simulink model "induction_motor_simplified_dynamic_model_pu"  (Simulink 7.5)
settings: Solver=ode45  StartTime=0.0  StopTime=2  MaxStep=100e-6  RelTol=1e-3
InitFcn:
  | clc;
  | clear;
  | 
  | f=50;          % motor supply frequency
  | Rs=0.01;     % Stator resistance in pu
  | Rr=0.02;     % Rotor resistance in pu
  | Lls=0.10;     % Stator leakage inductance in pu
  | Llr=0.10;     % Rotor leakage inductance in pu
  | Lm=4.50;    % Magnetising reactance in pu
  | wb=2*pi*f;  % base frequency
StopFcn:
  | figure(1);
  | plot(wm,Te,'-r');
  | grid;
  | title('Torque-speed X-tics');
  | xlabel('Speed [pu]');
  | ylabel('Torque [pu]');
  | clear;
libraries: powerlib x1
Description:
  | Mathematical model of the induction machine described in the rotor flux
  | reference frame.(Per unit formulation)
  | 
  |  Electrical  system equations:
  | 
  |  Vs = Rs is + (1/wb) (dfs/dt) + wf M(pi/2) fs
  | 
  |  where the variables is, vs, and fs are 2-dimensional space vectors
  |  and M(pi/2) represents a 90 degree space rotator namely  [0 -1;1 0]
  | 
  | wf = wm + wr;
  | wr = Rr Lm/Lr (iqs / fdr)
  | 1/wb Lr/Rr (dfdr/dt) + fdr = Lm ids
  | fqr = 0
  | 
  | The flux linkage current relations:
  | fs = Ls is + Lm ir
  | fr = Lm is  + Lr ir
  | Ls= Lm + Lls;
  | Lr = Lm + Lrl
  | 
  | Mechanical system equations:
  | Te = 2H (dwm/dt) + Bm wm + Tl
  | where Te = Lm/Lr (iqs fdr)
settings Model: Creator=Abdul Rahman Kashif  LastModifiedBy=Abdul Rahman Kashif
settings DataIOCC: LimitDataPoints=off  OutputSaveName=wm,Te

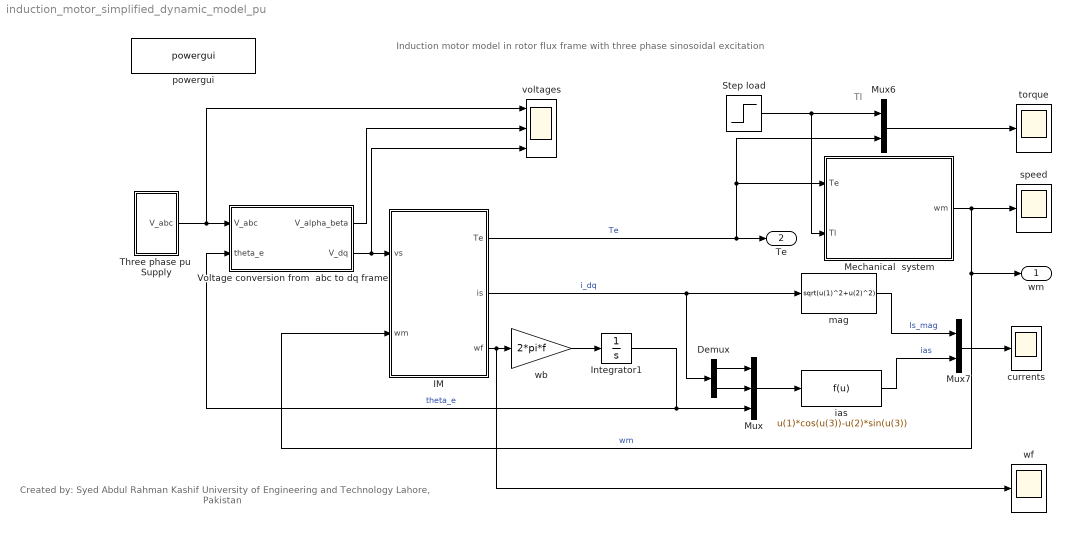
== system induction_motor_simplified_dynamic_model_pu ==
  note: Tl
  note: Induction motor model in rotor flux frame with three phase sinosoidal excitation
  note: Created by: Syed Abdul Rahman Kashif
      | University of Engineering and Technology
      | Lahore, Pakistan
  Demux : Demux  Outputs=2
  IM : Subsystem
  Integrator1 : Integrator
  Mechanical  system : Subsystem  mask{H=0.30, Bm=1e-5}
      mask prompts: H "Inertia constant [s]"; Bm "Damping coefficient [pu]"
      mask Display: disp('Mechanical\nSystem')
  Mux : Mux  Inputs=3
  Mux6 : Mux  Inputs=2
  Mux7 : Mux  Inputs=2
  Step load : Step  Time=1.5  Before=0.0  SampleTime=0
  Three phase pu  Supply : Subsystem  mask{f=f}
      mask prompts: f "Frequency"
  Voltage conversion from  abc to dq frame : Subsystem
  currents : Scope
      settings: TimeRange=2  YMin=-6  YMax=10  SaveName=ScopeData3
  ias : Fcn  Expr=u(1)*cos(u(3))-u(2)*sin(u(3))
  mag : Fcn  Expr=sqrt(u(1)^2+u(2)^2)
  powergui : powerlib/powergui  Priority=1  SystemSampleTime=-1  SimulationMode=Continuous  SampleTime=5e-6  frequency=60  SPID=off  DisableSnubberDevices=off  DisableRonSwitches=off  DisableVfSwitches=off  SwTol=0  Interpol=off  frequencyindice=50  echomessages=off  HookPort=off  DisplayEquations=off  FunctionMessages=off  EnableUseOfTLC=off  x0status=blocks  RestoreLinks=warning  ResistiveCurrentMeasurement=off  Frange=[0:2:500]  Ylog=off  Xlog=on  ShowGrid=off  save=off  variable=ZData  ZoomFFT=on  StartTime=0.0  cycles=1  DisplayStyle=1  fundamental=60  FreqAxis=off  MaxFrequency=1000  frequencyindicesteady=1  RmsSteady=1  display=off  Ts=0  methode=off
  speed : Scope
      settings: TimeRange=2  YMin=0  YMax=1.4  SaveName=wm  MaxDataPoints=20000  Decimation=20
  torque : Scope
      settings: TimeRange=2  YMin=-3  YMax=3  MaxDataPoints=20000  Decimation=20
  voltages : Scope  NumInputPorts=3
      settings: TimeRange=0.02  YMin=-1.5~-1.5~-0.5  YMax=1.5~1.5~1.5  SaveName=ScopeData2
  wb : Gain  Gain=2*pi*f  ParameterDataType=sfix(16)  ParameterScaling=2^0  OutDataType=sfix(16)  OutScaling=2^0  SaturateOnIntegerOverflow=on  OutDataTypeStr=Inherit: Same as input  ParamDataTypeStr=Inherit: Same as input
  wf : Scope
      settings: TimeRange=2  YMin=-2.5  YMax=2  MaxDataPoints=20000  Decimation=20
  wm : Outport
  Te : Outport  Port=2
  wires:
  Mux6/1 -> torque/1
  Mechanical  system/1(wm) -> speed/1, wm/1, IM/2(wm)  "wm"
  Voltage conversion from  abc to dq frame/2(V_dq) -> IM/1(vs), voltages/3
  Step load/1 -> Mux6/1, Mechanical  system/2(Tl)
  Demux/1 -> Mux/1
  Demux/2 -> Mux/2
  Mux/1 -> ias/1
  ias/1 -> Mux7/2  "ias"
  mag/1 -> Mux7/1  "Is_mag"
  Mux7/1 -> currents/1
  IM/2(is) -> mag/1, Demux/1  "i_dq"
  IM/1(Te) -> Te/1, Mux6/2, Mechanical  system/1(Te)  "Te"
  wb/1 -> Integrator1/1
  IM/3(wf) -> wb/1, wf/1
  Integrator1/1 -> Mux/3, Voltage conversion from  abc to dq frame/2(theta_e)  "theta_e"
  Voltage conversion from  abc to dq frame/1(V_alpha_beta) -> voltages/2
  Three phase pu  Supply/1(V_abc) -> voltages/1, Voltage conversion from  abc to dq frame/1(V_abc)

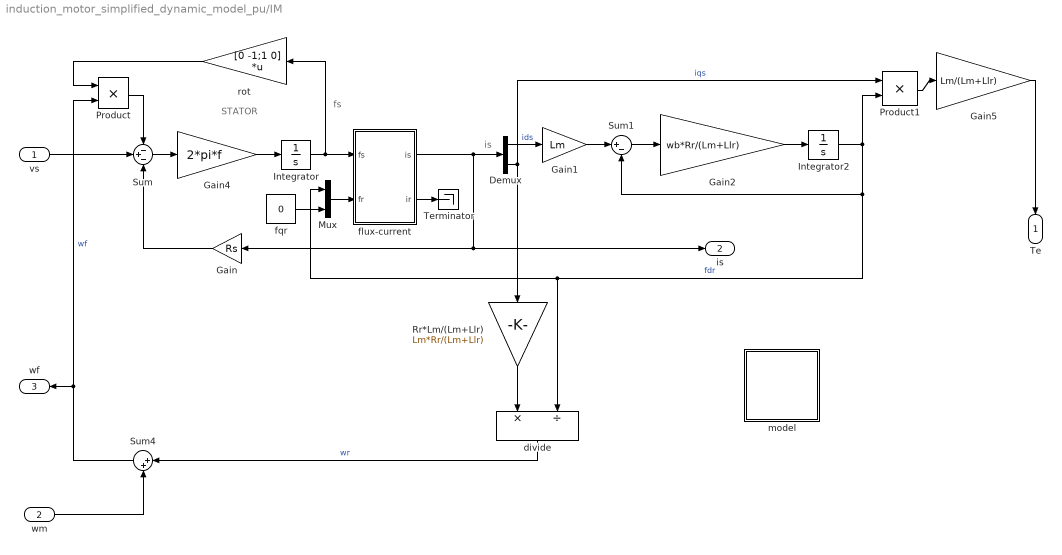
== system induction_motor_simplified_dynamic_model_pu/IM ==
  note: STATOR
  note: fs
  note: is
  vs : Inport  OutDataType=sfix(16)  OutScaling=2^0
  wm : Inport  Port=2  OutDataType=sfix(16)  OutScaling=2^0
  Demux : Demux  Outputs=2
  Gain : Gain  Gain=Rs  ParameterDataType=sfix(16)  ParameterScaling=2^0  OutDataType=sfix(16)  OutScaling=2^0  SaturateOnIntegerOverflow=on  OutDataTypeStr=Inherit: Same as input  ParamDataTypeStr=Inherit: Same as input
  Gain1 : Gain  Gain=Lm  ParameterDataType=sfix(16)  ParameterScaling=2^0  OutDataType=sfix(16)  OutScaling=2^0  SaturateOnIntegerOverflow=on  OutDataTypeStr=Inherit: Same as input  ParamDataTypeStr=Inherit: Same as input
  Gain2 : Gain  Gain=wb*Rr/(Lm+Llr)  ParameterDataType=sfix(16)  ParameterScaling=2^0  OutDataType=sfix(16)  OutScaling=2^0  SaturateOnIntegerOverflow=on  OutDataTypeStr=Inherit: Same as input  ParamDataTypeStr=Inherit: Same as input
  Gain4 : Gain  Gain=2*pi*f  ParameterDataType=sfix(16)  ParameterScaling=2^0  OutDataType=sfix(16)  OutScaling=2^0  SaturateOnIntegerOverflow=on  OutDataTypeStr=Inherit: Same as input  ParamDataTypeStr=Inherit: Same as input
  Gain5 : Gain  Gain=Lm/(Lm+Llr)  ParameterDataType=sfix(16)  ParameterScaling=2^0  OutDataType=sfix(16)  OutScaling=2^0  SaturateOnIntegerOverflow=on  OutDataTypeStr=Inherit: Same as input  ParamDataTypeStr=Inherit: Same as input
  Integrator : Integrator  InitialCondition=[0 0]
  Integrator2 : Integrator  InitialCondition=1e-5
  Mux : Mux  Inputs=2
  Product : Product  OutDataType=sfix(16)  OutScaling=2^0  SaturateOnIntegerOverflow=on  InputSameDT=on  OutDataTypeStr=Inherit: Same as first input
  Product1 : Product  OutDataType=sfix(16)  OutScaling=2^0  SaturateOnIntegerOverflow=on  InputSameDT=on  OutDataTypeStr=Inherit: Same as first input
  Rr*Lm/(Lm+Llr) : Gain  Gain=Lm*Rr/(Lm+Llr)  ParameterDataType=sfix(16)  ParameterScaling=2^0  OutDataType=sfix(16)  OutScaling=2^0  SaturateOnIntegerOverflow=on  OutDataTypeStr=Inherit: Same as input  ParamDataTypeStr=Inherit: Same as input
  Sum : Sum  Inputs=-+-  OutDataType=sfix(16)  OutScaling=2^0  SaturateOnIntegerOverflow=on  InputSameDT=on  OutDataTypeStr=Inherit: Same as first input
  Sum1 : Sum  Inputs=|+-  OutDataType=sfix(16)  OutScaling=2^0  SaturateOnIntegerOverflow=on  InputSameDT=on  OutDataTypeStr=Inherit: Same as first input
  Sum4 : Sum  Inputs=|++  OutDataType=sfix(16)  OutScaling=2^0  SaturateOnIntegerOverflow=on  InputSameDT=on  OutDataTypeStr=Inherit: Same as first input
  Terminator : Terminator
  divide : Product  Inputs=*/  OutDataType=sfix(16)  OutScaling=2^0  SaturateOnIntegerOverflow=on  InputSameDT=on  OutDataTypeStr=Inherit: Same as first input
  flux-current : Subsystem
  fqr : Constant  Value=0  OutDataType=sfix(16)  OutScaling=2^0
  model : Subsystem
      mask Display:
      | plot(-1.5,-1.5,1.5,1.5,cos(0:.01:7),sin(0:.01:7) )
      | disp('MODEL')
  rot : Gain  Gain=[0 -1;1 0]  Multiplication=Matrix(K*u)  ParameterDataType=sfix(16)  ParameterScaling=2^0  OutDataType=sfix(16)  OutScaling=2^0  SaturateOnIntegerOverflow=on  OutDataTypeStr=Inherit: Same as input  ParamDataTypeStr=Inherit: Same as input
  Te : Outport
  is : Outport  Port=2
  wf : Outport  Port=3
  wires:
  Gain/1 -> Sum/3
  Integrator/1 -> flux-current/1(fs), rot/1
  Product/1 -> Sum/1
  rot/1 -> Product/1
  Sum/1 -> Gain4/1
  Gain4/1 -> Integrator/1
  flux-current/1(is) -> Gain/1, is/1, Demux/1
  vs/1 -> Sum/2
  wm/1 -> Sum4/2
  Rr*Lm/(Lm+Llr)/1 -> divide/1
  Demux/1 -> Gain1/1  "ids"
  Sum4/1 -> Product/2, wf/1  "wf"
  divide/1 -> Sum4/1  "wr"
  fqr/1 -> Mux/2
  Demux/2 -> Rr*Lm/(Lm+Llr)/1, Product1/1  "iqs"
  Gain1/1 -> Sum1/1
  Sum1/1 -> Gain2/1
  Gain2/1 -> Integrator2/1
  Integrator2/1 -> divide/2, Mux/1, Sum1/2, Product1/2  "fdr"
  Product1/1 -> Gain5/1
  Gain5/1 -> Te/1
  Mux/1 -> flux-current/2(fr)
  flux-current/2(ir) -> Terminator/1

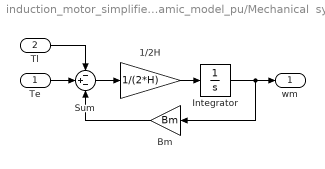
== system induction_motor_simplified_dynamic_model_pu/Mechanical  system ==
  Te : Inport  OutDataType=sfix(16)  OutScaling=2^0
  Tl : Inport  Port=2  OutDataType=sfix(16)  OutScaling=2^0
  1/2H : Gain  Gain=1/(2*H)  ParameterDataType=sfix(16)  ParameterScaling=2^0  OutDataType=sfix(16)  OutScaling=2^0  SaturateOnIntegerOverflow=on  OutDataTypeStr=Inherit: Same as input  ParamDataTypeStr=Inherit: Same as input
  Bm : Gain  Gain=Bm  ParameterDataType=sfix(16)  ParameterScaling=2^0  OutDataType=sfix(16)  OutScaling=2^0  SaturateOnIntegerOverflow=on  OutDataTypeStr=Inherit: Same as input  ParamDataTypeStr=Inherit: Same as input
  Integrator : Integrator
  Sum : Sum  Inputs=-+-  OutDataType=sfix(16)  OutScaling=2^0  SaturateOnIntegerOverflow=on  InputSameDT=on  OutDataTypeStr=Inherit: Same as first input
  wm : Outport
  wires:
  1/2H/1 -> Integrator/1
  Sum/1 -> 1/2H/1
  Bm/1 -> Sum/3
  Integrator/1 -> Bm/1, wm/1
  Te/1 -> Sum/2
  Tl/1 -> Sum/1

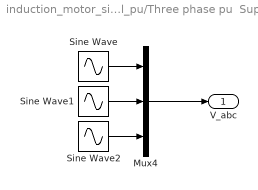
== system induction_motor_simplified_dynamic_model_pu/Three phase pu  Supply ==
  Mux4 : Mux  Inputs=3
  Sine Wave : Sin  Amplitude=1  Bias=0  Frequency=2*pi*f  Phase=pi  Samples=10  SampleTime=0  Offset=0
  Sine Wave1 : Sin  Amplitude=1  Bias=0  Frequency=2*pi*f  Phase=pi-2*pi/3  Samples=10  SampleTime=0  Offset=0
  Sine Wave2 : Sin  Amplitude=1  Bias=0  Frequency=2*pi*f  Phase=pi+2*pi/3  Samples=10  SampleTime=0  Offset=0
  V_abc : Outport
  wires:
  Sine Wave/1 -> Mux4/1
  Sine Wave1/1 -> Mux4/2
  Sine Wave2/1 -> Mux4/3
  Mux4/1 -> V_abc/1

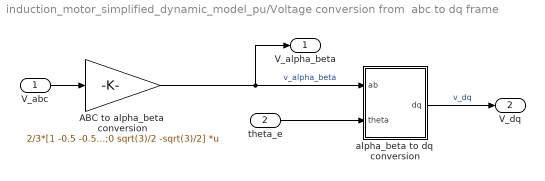
== system induction_motor_simplified_dynamic_model_pu/Voltage conversion from  abc to dq frame ==
  V_abc : Inport
  theta_e : Inport  Port=2
  ABC to alpha_beta  conversion : Gain  Gain=2/3*[1 -0.5 -0.5;0 sqrt(3)/2 -sqrt(3)/2]  Multiplication=Matrix(K*u)  ParameterDataType=sfix(16)  ParameterScaling=2^0  OutDataType=sfix(16)  OutScaling=2^0  SaturateOnIntegerOverflow=on  OutDataTypeStr=Inherit: Same as input  ParamDataTypeStr=Inherit: Same as input
  alpha_beta to dq  conversion : Subsystem
  V_alpha_beta : Outport
  V_dq : Outport  Port=2
  wires:
  ABC to alpha_beta  conversion/1 -> alpha_beta to dq  conversion/1(ab), V_alpha_beta/1  "v_alpha_beta"
  V_abc/1 -> ABC to alpha_beta  conversion/1
  theta_e/1 -> alpha_beta to dq  conversion/2(theta)
  alpha_beta to dq  conversion/1(dq) -> V_dq/1  "v_dq"

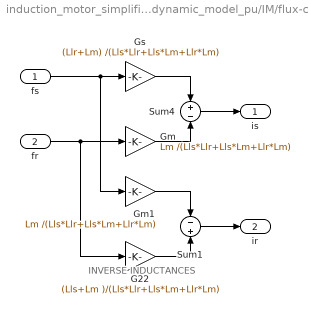
== system induction_motor_simplified_dynamic_model_pu/IM/flux-current ==
  note: INVERSE INDUCTANCES
  fs : Inport  OutDataType=sfix(16)  OutScaling=2^0
  fr : Inport  Port=2  OutDataType=sfix(16)  OutScaling=2^0
  G22 : Gain  Gain=(Lls+Lm )/(Lls*Llr+Lls*Lm+Llr*Lm)  ParameterDataType=sfix(16)  ParameterScaling=2^0  OutDataType=sfix(16)  OutScaling=2^0  SaturateOnIntegerOverflow=on  OutDataTypeStr=Inherit: Same as input  ParamDataTypeStr=Inherit: Same as input
  Gm : Gain  Gain=Lm /(Lls*Llr+Lls*Lm+Llr*Lm)  ParameterDataType=sfix(16)  ParameterScaling=2^0  OutDataType=sfix(16)  OutScaling=2^0  SaturateOnIntegerOverflow=on  OutDataTypeStr=Inherit: Same as input  ParamDataTypeStr=Inherit: Same as input
  Gm1 : Gain  Gain=Lm /(Lls*Llr+Lls*Lm+Llr*Lm)  ParameterDataType=sfix(16)  ParameterScaling=2^0  OutDataType=sfix(16)  OutScaling=2^0  SaturateOnIntegerOverflow=on  OutDataTypeStr=Inherit: Same as input  ParamDataTypeStr=Inherit: Same as input
  Gs : Gain  Gain=(Llr+Lm) /(Lls*Llr+Lls*Lm+Llr*Lm)  ParameterDataType=sfix(16)  ParameterScaling=2^0  OutDataType=sfix(16)  OutScaling=2^0  SaturateOnIntegerOverflow=on  OutDataTypeStr=Inherit: Same as input  ParamDataTypeStr=Inherit: Same as input
  Sum1 : Sum  Inputs=-+  OutDataType=sfix(16)  OutScaling=2^0  SaturateOnIntegerOverflow=on  InputSameDT=on  OutDataTypeStr=Inherit: Same as first input
  Sum4 : Sum  Inputs=+-  OutDataType=sfix(16)  OutScaling=2^0  SaturateOnIntegerOverflow=on  InputSameDT=on  OutDataTypeStr=Inherit: Same as first input
  is : Outport
  ir : Outport  Port=2
  wires:
  fs/1 -> Gs/1, Gm1/1
  Gs/1 -> Sum4/1
  fr/1 -> Gm/1, G22/1
  Gm/1 -> Sum4/2
  Sum4/1 -> is/1
  Gm1/1 -> Sum1/1
  G22/1 -> Sum1/2
  Sum1/1 -> ir/1

== system induction_motor_simplified_dynamic_model_pu/IM/model ==
  note: Mathematical model of the induction machine
      | described in the rotor flux reference frame.
      | (Per unit formulation)
  note: Electrical  system equations:
      |             vs = Rs is + 1/wo (dfs/dt) + wf M(pi/2) fs
      |                   where the variables is, vs, and fs are 2-dimensional space vectors
      |                   and M(pi/2) represents a 90o space rotator namely  [0 -1;1 0]
      |             wf = wm + wr;  wr = Rr Lm/Lr (iqs / fdr)
      |              1/wo Lr/Rr (dfdr/dt) + fdr = Lm ids
      |              fqr = 0
      |
      |  The flux linkage current relations :
      |           fs = Ls is + Lm ir
      |           fr =  Lm is  + Lr ir
      |                           Ls= Lm + Lsl  ;  Lr = Lm + Lrl
      |
      |   Mechanical system equations:
      |              Te = 2H (dwm/dt) + Bm wm + Tl
      |             where Te = Lm/Lr (iqs fdr)

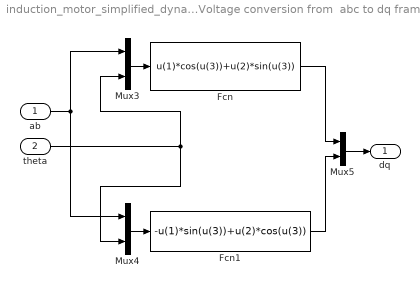
== system induction_motor_simplified_dynamic_model_pu/Voltage conversion from  abc to dq frame/alpha_beta to dq  conversion ==
  ab : Inport  OutDataType=sfix(16)  OutScaling=2^0
  theta : Inport  Port=2  OutDataType=sfix(16)  OutScaling=2^0
  Fcn : Fcn  Expr=u(1)*cos(u(3))+u(2)*sin(u(3))
  Fcn1 : Fcn  Expr=-u(1)*sin(u(3))+u(2)*cos(u(3))
  Mux3 : Mux  Inputs=2
  Mux4 : Mux  Inputs=2
  Mux5 : Mux  Inputs=2
  dq : Outport
  wires:
  Mux3/1 -> Fcn/1
  Mux4/1 -> Fcn1/1
  ab/1 -> Mux3/1, Mux4/1
  theta/1 -> Mux3/2, Mux4/2
  Fcn1/1 -> Mux5/2
  Fcn/1 -> Mux5/1
  Mux5/1 -> dq/1
